simulink model "quantization_sim"  (Simulink 8.3)
settings: Solver=ode5  StartTime=0.0  StopTime=1  FixedStep=1/8000  RelTol=1e-3
values from neighbouring files (symbols this model uses):
  freq = 1    [quantization_si.m]
  sourceAmp = A(k)    [quantization_si.m]
libraries: commutil2 x2, commsrccod2 x2, dspstat3 x1
settings Model: Creator=hlzhang  LastModifiedBy=hlzhang
settings DataIOCC: SignalLoggingName=sigsOut
settings DebuggingCC: SaveWithParameterizedLinksMsg=none  SignalResolutionControl=TryResolveAllWithWarning  SolverPrmCheckMsg=none  MultiTaskDSMMsg=warning  MultiTaskCondExecSysMsg=none  StateNameClashWarn=none  StrictBusMsg=None
settings HardwareCC: TargetUnknown=on
settings RTWCC: IncludeERTFirstTime=on

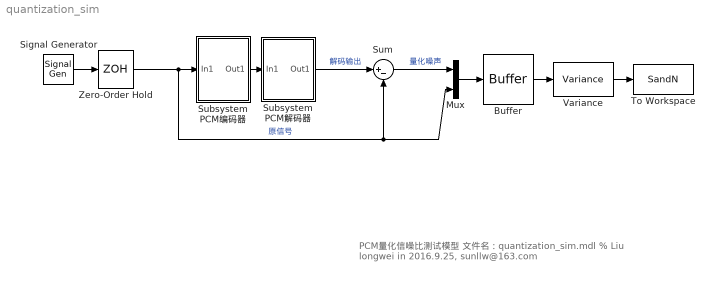
== system quantization_sim ==
  note: PCM量化信噪比测试模型
      | 文件名：quantization_sim.mdl
      | % Liu longwei in 2016.9.25, sunllw@163.com
  Buffer : Buffer  N=8000  ic=1
  Mux : Mux  Inputs=2
  Signal Generator : SignalGenerator  Amplitude=sourceAmp  Frequency=freq
  Subsystem PCM编码器 : Subsystem
  Subsystem PCM解码器 : Subsystem
  Sum : Sum  Inputs=|+-  SaturateOnIntegerOverflow=on
  To Workspace : ToWorkspace  VariableName=SandN  SampleTime=-1
      settings: MaxDataPoints=1
  Variance : dspstat3/Variance  run=off  reset_popup=None  InputProcessing=Columns as channels (frame based)  directionMode=Each column  dimension=1  treatSBRowAsCol=on  roiEnable=off  roiType=Rectangles  roiPortion=Entire ROI  roiOutput=Individual statistics for each ROI  roiFlag=off  roundingMode=Floor  overflowMode=off
  Zero-Order Hold : ZeroOrderHold  SampleTime=1/8000
  wires:
  Signal Generator/1 -> Zero-Order Hold/1
  Subsystem PCM编码器/1(Out1) -> Subsystem PCM解码器/1(In1)
  Zero-Order Hold/1 -> Subsystem PCM编码器/1(In1), Mux/2, Sum/2  "原信号"
  Subsystem PCM解码器/1(Out1) -> Sum/1  "解码输出"
  Mux/1 -> Buffer/1
  Buffer/1 -> Variance/1
  Variance/1 -> To Workspace/1
  Sum/1 -> Mux/1  "量化噪声"

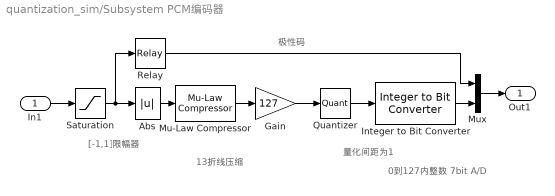
== system quantization_sim/Subsystem PCM编码器 ==
  note: 0到127内整数
      | 7bit A/D
  note: [-1,1]限幅器
  note: 极性码
  note: 13折线压缩
  note: 量化间距为1
  In1 : Inport
  Abs : Abs  SaturateOnIntegerOverflow=on
  Gain : Gain  Gain=127  SaturateOnIntegerOverflow=on  OutDataTypeStr=Inherit: Same as input  ParamDataTypeStr=Inherit: Same as input
  Integer to Bit Converter : commutil2/Integer to Bit Converter  nbits=7
  Mu-Law Compressor : commsrccod2/Mu-Law Compressor  mu=mu  V=1
  Mux : Mux  Inputs=2
  Quantizer : Quantizer  QuantizationInterval=1
  Relay : Relay
  Saturation : Saturate  UpperLimit=1  LowerLimit=-1
  Out1 : Outport
  wires:
  Mu-Law Compressor/1 -> Gain/1
  Quantizer/1 -> Integer to Bit Converter/1
  Gain/1 -> Quantizer/1
  Abs/1 -> Mu-Law Compressor/1
  Relay/1 -> Mux/1
  Integer to Bit Converter/1 -> Mux/2
  Saturation/1 -> Abs/1, Relay/1
  Mux/1 -> Out1/1
  In1/1 -> Saturation/1

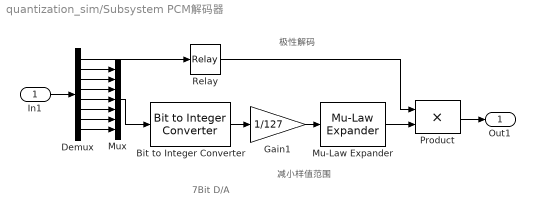
== system quantization_sim/Subsystem PCM解码器 ==
  note: 极性解码
  note: 7Bit D/A
  note: 减小样值范围
  In1 : Inport
  Bit to Integer Converter : commutil2/Bit to Integer Converter  nbits=7  bitOrder=MSB first  signedOutputValues=Unsigned  outDtype=Inherit via internal rule  outDtypeSigned=Inherit via internal rule
  Demux : Demux  Outputs=8
  Gain1 : Gain  Gain=1/127  SaturateOnIntegerOverflow=on  OutDataTypeStr=Inherit: Same as input  ParamDataTypeStr=Inherit: Same as input
  Mu-Law Expander : commsrccod2/Mu-Law Expander  mu=mu  V=1
  Mux : Mux  Inputs=7
  Product : Product  SaturateOnIntegerOverflow=on  OutDataTypeStr=Inherit: Same as first input
  Relay : Relay  OnSwitchValue=0.5  OffSwitchValue=0.5  OffOutputValue=-1
  Out1 : Outport
  wires:
  Bit to Integer Converter/1 -> Gain1/1
  Mu-Law Expander/1 -> Product/2
  Relay/1 -> Product/1
  Mux/1 -> Bit to Integer Converter/1
  Demux/1 -> Relay/1
  Demux/2 -> Mux/1
  Demux/3 -> Mux/2
  Demux/8 -> Mux/7
  Demux/7 -> Mux/6
  Demux/6 -> Mux/5
  Demux/5 -> Mux/4
  Demux/4 -> Mux/3
  Gain1/1 -> Mu-Law Expander/1
  In1/1 -> Demux/1
  Product/1 -> Out1/1
